simulink model "rlc_circuit"  (R2021a)
settings: Solver=VariableStepAuto  StartTime=0.0  StopTime=0.05  MaxStep=0.000001  RelTol=1e-3
values from neighbouring files (symbols this model uses):
  A = adj    [ceren_function.m]    (also in deneme.m = [-resi/L -1/L; 1/C 0]; get_mass_spring_model.m = [0 1 0 0; (-k1-k2)/m1 0 k2/m1 0; 0 0 0 1; k2/m2 0 -k2/m2 0]; matlab.mat = [0  -100; 1000  0])
  B = [1/L; 0]    [deneme.m]    (also in get_mass_spring_model.m = [0; 1/m1; 0; 0]; matlab.mat = [100 0])
  C = [0 1]    [deneme.m]    (also in get_mass_spring_model.m = [1 0 0 0; 0 0 1 0]; matlab.mat)
  c = 200    [init_graph.m]    (also in matlab.mat = 10)
  D = [0]    [deneme.m]    (also in get_mass_spring_model.m = [0; 0; 0;0]; matlab.mat = 0)
  K = [7.50549770549 2.31662479036]    [matlab.mat]
settings Model: PacingRate=9  Creator=umut  LastModifiedBy=umut
settings DebuggingCC: UnderSpecifiedDimensionMsg=warning

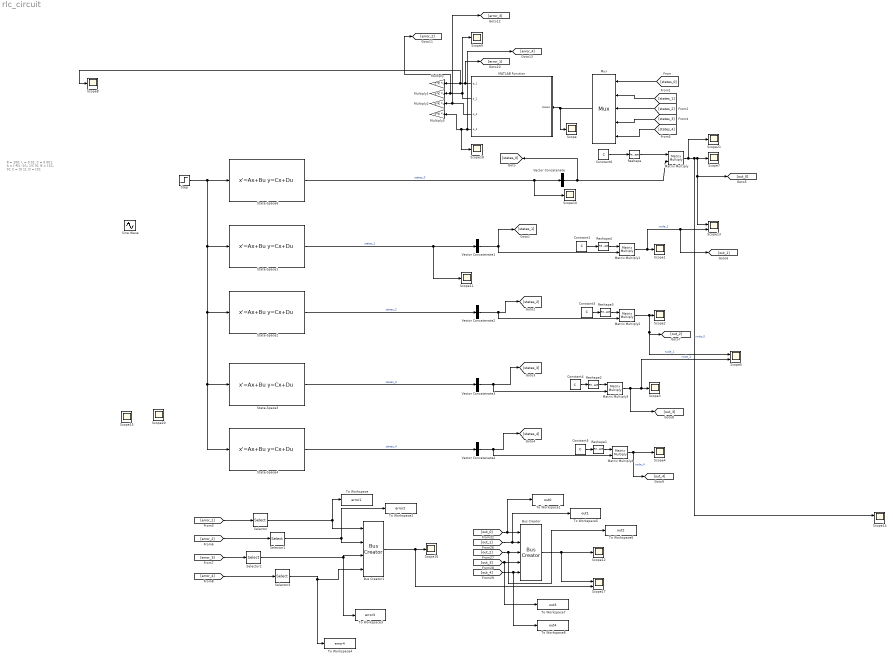
== system rlc_circuit ==
  note: R = 100;
      | L = 0.01;
      | C =  0.001;
      |
      | A = [-R/L -1/L; 1/C 0];
      | B = [1/L; 0];
      | C = [0 1];
      | D = [0];
  Bus Creator : BusCreator  Inputs=5
  Bus Creator1 : BusCreator  Inputs=4
  Constant{1,3..6} (5 alike) : Constant  Value=C
  MATLAB Function : MATLAB Function  TreatAsAtomicUnit=on
  Matrix Multiply{,1..4} (5 alike) : Product  Multiplication=Matrix(*)
  Multiply{,1..3} (4 alike) : Gain  Gain=c*K  Multiplication=Matrix(K*u)
  Mux : Mux  Inputs=5
  Reshape{,1..4} (5 alike) : Reshape  OutputDimensionality=Customize  OutputDimensions=[1,2]
  Scope{,1..4,7..12,15..16,18,20..21} (16 alike) : Scope
  Scope{5,13..14,17} (4 alike) : Scope  NumInputPorts=2
  Selector{,1..3} (4 alike) : Selector  InputPortWidth=2  IndexOptions=Starting index (dialog)  Indices=2  OutputSizes=1
  Sine Wave : Sin  SampleTime=0
  State-Space1 : StateSpace  A=A  B=B  C=eye(2)  D=[D;D]  InitialCondition=[30;80]
  State-Space2 : StateSpace  A=A  B=B  C=eye(2)  D=[D;D]  InitialCondition=[30;100]
  State-Space3 : StateSpace  A=A  B=B  C=eye(2)  D=[D;D]  InitialCondition=[20;60]
  State-Space4 : StateSpace  A=A  B=B  C=eye(2)  D=[D;D]  InitialCondition=[20;40]
  State-Space6 : StateSpace  A=A  B=B  C=eye(2)  D=[D;D]  InitialCondition=[20;0]
  Step : Step  After=0  SampleTime=0
  To Workspace : ToWorkspace  VariableName=error1  SampleTime=-1
      settings: Save2DSignal=2-D array (concatenate along first dimension)
  To Workspace1 : ToWorkspace  VariableName=out0  SampleTime=-1
      settings: Save2DSignal=2-D array (concatenate along first dimension)
  To Workspace2 : ToWorkspace  VariableName=error2  SampleTime=-1
      settings: Save2DSignal=2-D array (concatenate along first dimension)
  To Workspace3 : ToWorkspace  VariableName=error3  SampleTime=-1
      settings: Save2DSignal=2-D array (concatenate along first dimension)
  To Workspace4 : ToWorkspace  VariableName=error4  SampleTime=-1
      settings: Save2DSignal=2-D array (concatenate along first dimension)
  To Workspace5 : ToWorkspace  VariableName=out1  SampleTime=-1
      settings: Save2DSignal=2-D array (concatenate along first dimension)
  To Workspace6 : ToWorkspace  VariableName=out2  SampleTime=-1
      settings: Save2DSignal=2-D array (concatenate along first dimension)
  To Workspace7 : ToWorkspace  VariableName=out3  SampleTime=-1
      settings: Save2DSignal=2-D array (concatenate along first dimension)
  To Workspace8 : ToWorkspace  VariableName=out4  SampleTime=-1
      settings: Save2DSignal=2-D array (concatenate along first dimension)
  Vector Concatenate : Concatenate  NumInputs=1  Mode=Multidimensional array  ConcatenateDimension=4
  Vector Concatenate{1..4} (4 alike) : Concatenate  NumInputs=1  Mode=Multidimensional array  ConcatenateDimension=2
  wires:
  Matrix Multiply1/1 -> [out_1], Scope13/2, Scope1/1  "node_1"
  State-Space1/1 -> Scope11/1, Vector Concatenate1/1  "states_1"
  Mux/1 -> Scope/1, MATLAB Function/1(states)
  State-Space2/1 -> Vector Concatenate2/1  "states_2"
  Matrix Multiply2/1 -> [out_2], Scope5/1, Scope2/1  "node_2"
  Matrix Multiply3/1 -> [out_3], Scope5/2, Scope3/1  "node_3"
  State-Space3/1 -> Vector Concatenate3/1  "states_3"
  Matrix Multiply4/1 -> [out_4], Scope4/1  "node_4"
  State-Space4/1 -> Vector Concatenate4/1  "states_4"
  [states_0] -> Mux/1
  [states_1] -> Mux/2
  [states_4] -> Mux/5
  [states_3] -> Mux/4
  [states_2] -> Mux/3
  MATLAB Function/1(e_1) -> [error_1], Scope8/1, Multiply/1
  MATLAB Function/2(e_2) -> Scope9/1, [error_2], Multiply1/1
  MATLAB Function/3(e_3) -> [error_3], Multiply2/1
  MATLAB Function/4(e_4) -> Scope18/1, Multiply3/1, [error_4]
  Constant6/1 -> Reshape/1
  State-Space6/1 -> Scope10/1, Vector Concatenate/1  "states_0"
  Vector Concatenate/1 -> [states_0], Matrix Multiply/2
  Matrix Multiply/1 -> Scope21/1, Scope14/1, [out_0], Scope13/1, Scope7/1  "node_0"
  Vector Concatenate1/1 -> Matrix Multiply1/2, [states_1]
  Vector Concatenate2/1 -> Matrix Multiply2/2, [states_2]
  Vector Concatenate3/1 -> Matrix Multiply3/2, [states_3]
  Vector Concatenate4/1 -> Matrix Multiply4/2, [states_4]
  Constant1/1 -> Reshape4/1
  Constant3/1 -> Reshape3/1
  Constant4/1 -> Reshape2/1
  Constant5/1 -> Reshape1/1
  Reshape/1 -> Matrix Multiply/1
  Reshape4/1 -> Matrix Multiply1/1
  Reshape3/1 -> Matrix Multiply2/1
  Reshape2/1 -> Matrix Multiply3/1
  Reshape1/1 -> Matrix Multiply4/1
  [out_1] -> To Workspace5/1, Bus Creator/2
  [out_2] -> To Workspace6/1, Bus Creator/3
  [out_0] -> To Workspace1/1, Bus Creator/1
  [out_4] -> To Workspace8/1, Bus Creator/5
  [out_3] -> To Workspace7/1, Bus Creator/4
  Bus Creator/1 -> Scope12/1, Scope17/1
  Bus Creator1/1 -> Scope16/1, Scope17/2
  [error_1] -> Selector/1
  [error_2] -> Selector1/1
  [error_3] -> Selector2/1
  [error_4] -> Selector3/1
  Step/1 -> State-Space4/1, State-Space3/1, State-Space2/1, State-Space1/1, State-Space6/1
  Selector1/1 -> Bus Creator1/2, To Workspace2/1
  Selector/1 -> Bus Creator1/1, To Workspace/1
  Selector2/1 -> Bus Creator1/3, To Workspace3/1
  Selector3/1 -> To Workspace4/1, Bus Creator1/4

== matlab function rlc_circuit/MATLAB Function ==
  data: states input size=[10, 1]; e_1 output size=[2, 1]; e_2 output size=[2, 1]; e_3 output size=[2, 1]; e_4 output size=[2, 1]
function [e_1, e_2, e_3, e_4]  = calculate_neighborhood_error(states)
    adj = [ 0	0	0	0
            1	0	0	0
            0	1	0	0
            0	0	1	0];
    
    pinnings = [1; 0; 0; 0];

    A = adj;
    G = pinnings;
    
    size_agents = 4;
    size_states = 2;
    
    error = zeros(size_states, size_agents);
    
    
    for i = 1 : size_agents
        error_temp = [0;0];
        for j = 1 : size_agents
            error_temp = error_temp + A(i, j) * (states((j)*2+1 : 2*(j+1)) - states((i)*2+1 : 2*(i+1)));
        end
        error_temp = error_temp + pinnings(i) * (states(1 : 2) - states((i)*2+1 : 2*(i+1)));
        error(:,i) = error_temp;
    end
    
    e_1 = error(:,1);
    e_2 = error(:,2);
    e_3 = error(:,3);
    e_4 = error(:,4);
end
